simulink subsystem "Lqr_Controller"  (R2022b)
settings: Solver=VariableStepAuto  StartTime=0.0  StopTime=10.0  RelTol=1e-3
values from neighbouring files (symbols this model uses):
  K = lqr(SYSC, Q, R)    [Lqr_Controller_Tune.m]
  Ki = 0    [Lqr_Controller_Tune.m]
  Nu = N(4:end)    [Lqr_Controller_Tune.m]
  Nx = N(1:3)    [Lqr_Controller_Tune.m]
undefined symbols (not defined in the file or in its folder): conv, DiscIntNeverNeededParam, uc
settings Model: Creator=giuliapegoraro  LastModifiedBy=giuliapegoraro

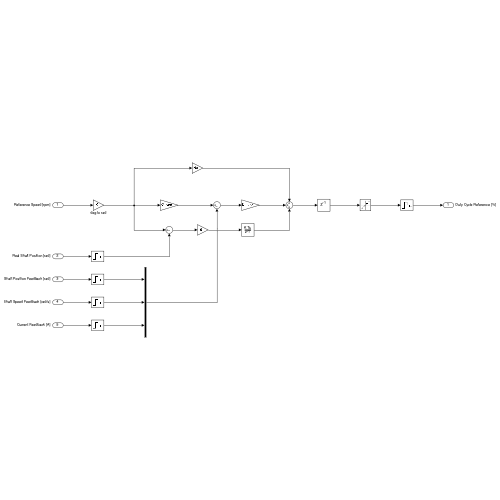
[thumbnail: Simulink's stored preview of the top-level diagram]
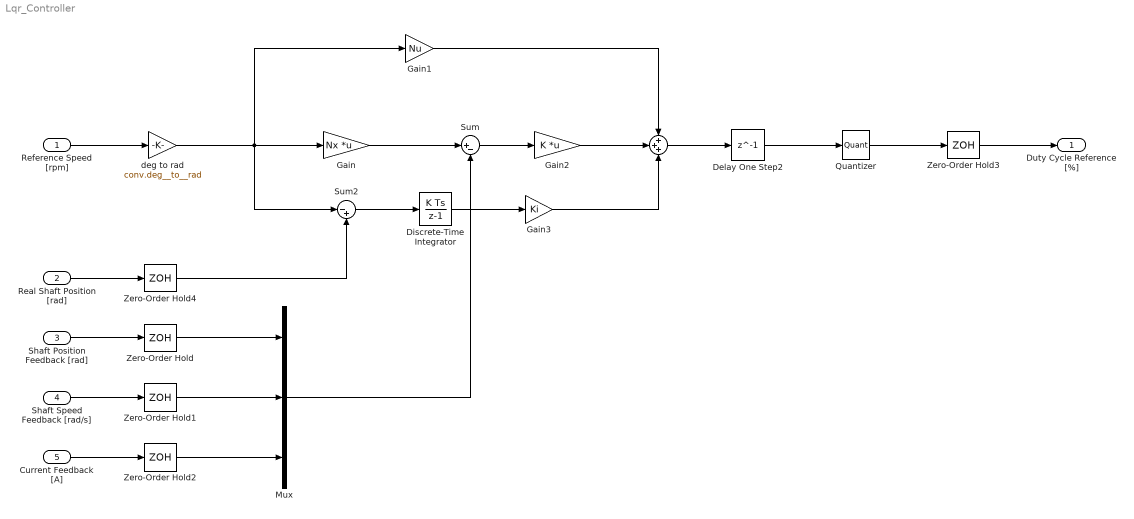
== system Lqr_Controller ==
  Reference Speed [rpm] : Inport
  Real Shaft Position [rad] : Inport  Port=2
  Shaft Position Feedback [rad] : Inport  Port=3
  Shaft Speed Feedback [rad/s] : Inport  Port=4
  Current Feedback [A] : Inport  Port=5
  " " : Sum  Inputs=+++
  Delay One Step2 : Delay  DelayLength=1
  Discrete-Time Integrator : DiscreteIntegrator  SampleTime=-1  ICPrevOutput=DiscIntNeverNeededParam  ICPrevScaledInput=DiscIntNeverNeededParam
  Gain : Gain  Gain=Nx  Multiplication=Matrix(K*u) (u vector)
  Gain1 : Gain  Gain=Nu
  Gain2 : Gain  Gain=K  Multiplication=Matrix(K*u) (u vector)
  Gain3 : Gain  Gain=Ki
  Mux : Mux  Inputs=3
  Quantizer : Quantizer  QuantizationInterval=uc.d_step
  Sum : Sum  Inputs=|+-
  Sum2 : Sum  Inputs=|-+
  Zero-Order Hold{,1..4} (5 alike) : ZeroOrderHold  SampleTime=uc.Ts
  deg to rad : Gain  Gain=conv.deg__to__rad
  Duty Cycle Reference [%] : Outport
  wires:
  Reference Speed [rpm]/1 -> deg to rad/1
  Shaft Position Feedback [rad]/1 -> Zero-Order Hold/1
  Shaft Speed Feedback [rad/s]/1 -> Zero-Order Hold1/1
  Current Feedback [A]/1 -> Zero-Order Hold2/1
  deg to rad/1 -> Sum2/1, Gain1/1, Gain/1
  Gain/1 -> Sum/1
  Sum/1 -> Gain2/1
  Gain2/1 -> " "/2
  Gain1/1 -> " "/1
  Zero-Order Hold1/1 -> Mux/2
  Zero-Order Hold/1 -> Mux/1
  Zero-Order Hold2/1 -> Mux/3
  Zero-Order Hold3/1 -> Duty Cycle Reference [%]/1
  Quantizer/1 -> Zero-Order Hold3/1
  " "/1 -> Delay One Step2/1
  Delay One Step2/1 -> Quantizer/1
  Real Shaft Position [rad]/1 -> Zero-Order Hold4/1
  Sum2/1 -> Discrete-Time Integrator/1
  Gain3/1 -> " "/3
  Zero-Order Hold4/1 -> Sum2/2
  Mux/1 -> Sum/2
  Discrete-Time Integrator/1 -> Gain3/1
